simulink model "SIL_CessnaC172"  (R2021b)
settings: Solver=FixedStepAuto  StartTime=0  StopTime=T  FixedStep=0.01  RelTol=1e-3  EnableMultiTasking=on
model workspace (MAT data in the model file):
  SL_ROS_VariableLengthArrays_MaxSizes.CommonInfo.ArrayTruncateAction = 'EmitWarning'
  SL_ROS_VariableLengthArrays_MaxSizes.MsgTypeMap = containers.Map
  SL_ROS_VariableLengthArrays_MaxSizes.MsgTypeMap.serialization.keys = {'aircraft_communication/NetworkComm', 'aircraft_messages/Communication', 'aircraft_messages/NetworkComm', 'sensor_msgs/Image'}
  SL_ROS_VariableLengthArrays_MaxSizes.MsgTypeMap.serialization.values{1}.PropertyName = 'Comms'
  SL_ROS_VariableLengthArrays_MaxSizes.MsgTypeMap.serialization.values{1}.DataType = 'aircraft_communication/Communication'
  SL_ROS_VariableLengthArrays_MaxSizes.MsgTypeMap.serialization.values{1}.MaxLength = 4
  SL_ROS_VariableLengthArrays_MaxSizes.MsgTypeMap.serialization.values{2}.PropertyName = 'Ssid'
  SL_ROS_VariableLengthArrays_MaxSizes.MsgTypeMap.serialization.values{2}.DataType = 'uint8'
  SL_ROS_VariableLengthArrays_MaxSizes.MsgTypeMap.serialization.values{2}.MaxLength = 6
  SL_ROS_VariableLengthArrays_MaxSizes.MsgTypeMap.serialization.values{3}.PropertyName = 'Comms'
  SL_ROS_VariableLengthArrays_MaxSizes.MsgTypeMap.serialization.values{3}.DataType = 'aircraft_messages/Communication'
  SL_ROS_VariableLengthArrays_MaxSizes.MsgTypeMap.serialization.values{3}.MaxLength = 4
  SL_ROS_VariableLengthArrays_MaxSizes.MsgTypeMap.serialization.values{4}(1).PropertyName = 'Data'
  SL_ROS_VariableLengthArrays_MaxSizes.MsgTypeMap.serialization.values{4}(1).DataType = 'uint8'
  SL_ROS_VariableLengthArrays_MaxSizes.MsgTypeMap.serialization.values{4}(1).MaxLength = 259200
  SL_ROS_VariableLengthArrays_MaxSizes.MsgTypeMap.serialization.values{4}(2).PropertyName = 'Encoding'
  SL_ROS_VariableLengthArrays_MaxSizes.MsgTypeMap.serialization.values{4}(2).DataType = 'uint8'
  SL_ROS_VariableLengthArrays_MaxSizes.MsgTypeMap.serialization.values{4}(2).MaxLength = 259200
  SL_ROS_VariableLengthArrays_MaxSizes.MsgTypeMap.serialization.uniformity = 0
  SL_ROS_VariableLengthArrays_MaxSizes.MsgTypeMap.serialization.keyType = 'char'
  SL_ROS_VariableLengthArrays_MaxSizes.MsgTypeMap.serialization.valueType = 'any'
values from neighbouring files (symbols this model uses):
  airspeed_ref = 42    [start_Cessna172.m]
  altitude_ref = 300    [start_Cessna172.m]
  N_Waypoints = size(Waypoints,1)    [start_Cessna172.m]
  radius_waypoint = 200    [start_Cessna172.m]
  Waypoints = [1000 -1000 ... (first row only)    [start_Cessna172.m]
undefined symbols (not defined in the file or in its folder): Elevators, Propeller, RightAileron, RightFlap, Rudder
libraries: robotlib x7, slpidlib x3
settings Model: Creator=fcsou  LastModifiedBy=fabricio
settings SolverCC: AlgebraicLoopSolver=TrustRegion
settings OptimizationCC: EnhancedBackFolding=on  PassReuseOutputArgsThreshold=0  MaxStackSize=64  OptimizeBlockOrder=speed  DifferentSizesBufferReuse=on  OptimizationCustomize=off
settings DebuggingCC: ParameterTunabilityLossMsg=error  SFMachineParentedDataDiag=warning
settings HardwareCC: ProdBitPerPointer=32  ProdBitPerSizeT=32  ProdBitPerPtrDiffT=32  ProdLargestAtomicFloat=None  ProdIntDivRoundTo=Undefined  ProdEndianess=Unspecified  ProdWordSize=32  ProdHWDeviceType=Generic->Unspecified (assume 32-bit Generic)  UseEmbeddedCoderFeatures=off
settings SFSimCC: MATLABDynamicMemAlloc=off
settings RTWCC: Description=Embedded Coder  SystemTargetFile=ert.tlc  HardwareBoard=Robot Operating System (ROS)  TLCOptions="-aInlineSetEventsForThisBaseRateFcn=TLC_FALSE -aSuppressMultiTaskScheduler=TLC_FALSE  -aRateBasedStepFcn=0"  TemplateMakefile=ert_default_tmf  Toolchain=Catkin  TargetLang=C++
settings CodeAppCC: ForceParamTrailComments=on  OperatorAnnotations=on
settings ERTTargetCC: ERTCustomFileBanners=off  SupportContinuousTime=on  SupportNonInlinedSFcns=on  RemoveResetFunc=off  ModelStepFunctionPrototypeControlCompliant=off  ERTCustomFileTemplate=rostime_codertarget_file_process.tlc

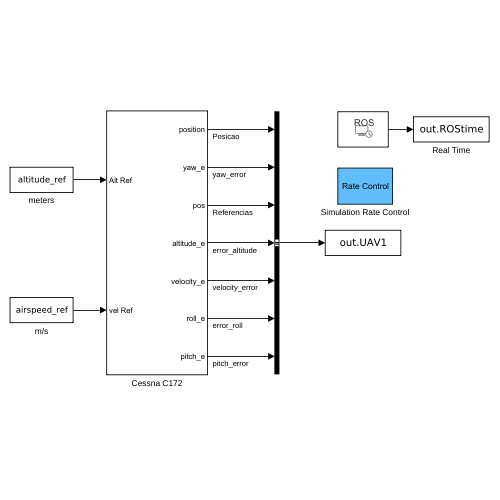
[thumbnail: Simulink's stored preview of the top-level diagram]
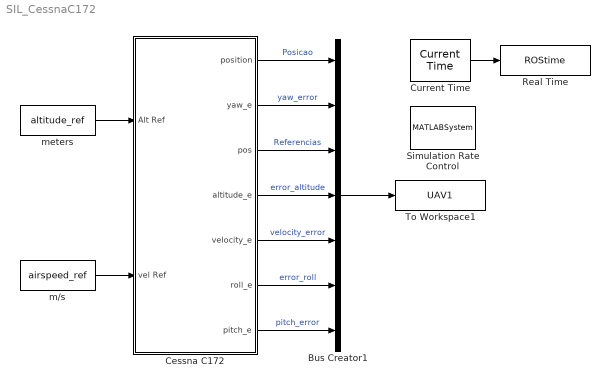
== system SIL_CessnaC172 ==
  Bus Creator1 : BusCreator  Inputs=7
  Cessna C172 : Subsystem
  Current Time : robotlib/Current Time  OutputFormat=double  SampleTime=-1  ModelName=SIL_CessnaC172
      settings: SourceProductBaseCode=RR
  Real Time : ToWorkspace  VariableName=ROStime  SaveFormat=Timeseries  SampleTime=-1
  Simulation Rate Control : MATLABSystem  System=ExampleHelperSimulationRateControl  SampleTime=0.01
      mask Type: ExampleHelperSimulationRateControl
      mask Display: disp('Rate Control');
  To Workspace1 : ToWorkspace  VariableName=UAV1  SaveFormat=Timeseries  SampleTime=-1
  m/s : Constant  Value=airspeed_ref
  meters : Constant  Value=altitude_ref
  wires:
  m/s/1 -> Cessna C172/2(vel Ref)
  meters/1 -> Cessna C172/1(Alt Ref)
  Bus Creator1/1 -> To Workspace1/1
  Current Time/1 -> Real Time/1
  Cessna C172/1(position) -> Bus Creator1/1  "Posicao"
  Cessna C172/2(yaw_e) -> Bus Creator1/2  "yaw_error"
  Cessna C172/3(pos) -> Bus Creator1/3  "Referencias"
  Cessna C172/4(altitude_e) -> Bus Creator1/4  "error_altitude"
  Cessna C172/5(velocity_e) -> Bus Creator1/5  "velocity_error"
  Cessna C172/6(roll_e) -> Bus Creator1/6  "error_roll"
  Cessna C172/7(pitch_e) -> Bus Creator1/7  "pitch_error"

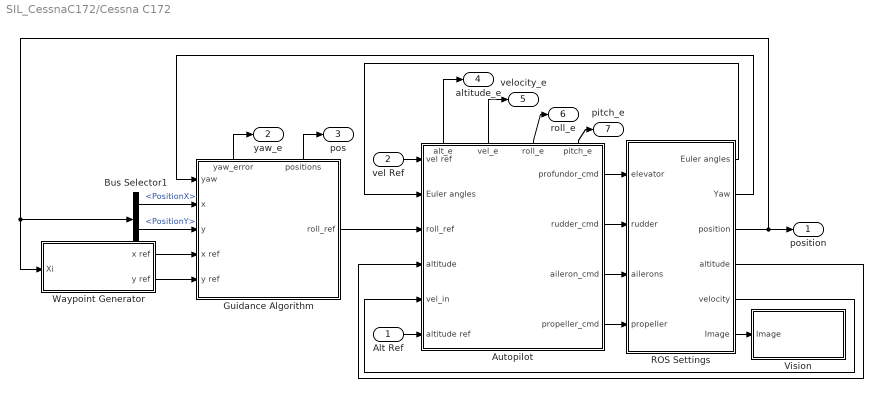
== system SIL_CessnaC172/Cessna C172 ==
  Alt Ref : Inport
  vel Ref : Inport  Port=2
  Autopilot : Subsystem
      settings: PortSchema="{\"entries\":[{\"content\":{\"sides\":[{\"content\":{\"connectorIds\":[\"In1\",\"In2\",\"In3\",\"In4\",\"In5\",\"In6\"]},\"type\":\"ConnectorPlacement.EquallySpacedRectSide\",\"uuid\":\"f5987fb5-26bd-460f-ada3-c62a2cc917d9\"},{\"content\":{\"connectorIds\":[\"Out1\",\"Out2\",\"Out3\",\"Out4\"],\"side\":\"RIGHT\"},\"type\":\"ConnectorPlacement.EquallySpacedRectSide\",\"uuid\":\"78b4fbb6-b2d6-45e8-a79e-ccfb1aa742fa\"},{\"content\":{\"connectorIds\":[\"Out5\",\"Out6\",\"Out7\",\"Out8\"],\"side\":\"TOP\"},\"type\":\"ConnectorPlacement.EquallySpacedRectSide\",\"uuid\":\"043ac8db-db42-42ba-ba46-d4f45f772f93\"},{\"content\":{\"connectorIds\":[],\"side\":\"HIDDEN\"},\"type\":\"ConnectorPlacement.EquallySpacedRectSide\",\"uuid\":\"557a5d68-6739-4613-818d-4b3751c4f08a\"}]},\"type\":\"ConnectorPlacement.EquallySpacedConnector\",\"uuid\":\"675ce67f-dd1b-4b16-8fb4-2c0be5e81414\"}],\"packageUris\":[\"http://schema.mathworks.com/mf0/Connector/R2020b\"],\"version\":\"1.0\"}"
  Bus Selector1 : BusSelector  OutputSignals=PositionX,PositionY
  Guidance Algorithm : Subsystem
      settings: PortSchema="{\"entries\":[{\"content\":{\"sides\":[{\"content\":{\"connectorIds\":[\"In1\",\"In2\",\"In3\",\"In4\",\"In5\"]},\"type\":\"ConnectorPlacement.EquallySpacedRectSide\",\"uuid\":\"b0b83658-dc10-4011-a234-ab17b261f867\"},{\"content\":{\"connectorIds\":[\"Out1\"],\"side\":\"RIGHT\"},\"type\":\"ConnectorPlacement.EquallySpacedRectSide\",\"uuid\":\"f99dae16-3a0a-4b7a-a248-8f98f89ef8fb\"},{\"content\":{\"connectorIds\":[\"Out2\",\"Out3\"],\"side\":\"TOP\"},\"type\":\"ConnectorPlacement.EquallySpacedRectSide\",\"uuid\":\"275bc05e-c915-4930-a6d1-ba5a3a506250\"},{\"content\":{\"connectorIds\":[],\"side\":\"HIDDEN\"},\"type\":\"ConnectorPlacement.EquallySpacedRectSide\",\"uuid\":\"a071ce22-c6e1-49a1-b318-d26a8e8cfe9f\"}]},\"type\":\"ConnectorPlacement.EquallySpacedConnector\",\"uuid\":\"e0998603-dd40-4b43-8488-1ee2e7350a27\"}],\"packageUris\":[\"http://schema.mathworks.com/mf0/Connector/R2020b\"],\"version\":\"1.0\"}"
  ROS Settings : Subsystem
  Vision : Subsystem
  Waypoint Generator : Subsystem
  position : Outport
  yaw_e : Outport  Port=2
  pos : Outport  Port=3
  altitude_e : Outport  Port=4
  velocity_e : Outport  Port=5
  roll_e : Outport  Port=6
  pitch_e : Outport  Port=7
  wires:
  Bus Selector1/2 -> Guidance Algorithm/3(y)  "<PositionY>"
  Bus Selector1/1 -> Guidance Algorithm/2(x)  "<PositionX>"
  Autopilot/3(aileron_cmd) -> ROS Settings/3(ailerons)
  ROS Settings/1(Euler angles) -> Autopilot/2(Euler angles)
  Guidance Algorithm/1(roll_ref) -> Autopilot/3(roll_ref)
  Autopilot/1(profundor_cmd) -> ROS Settings/1(elevator)
  ROS Settings/3(position) -> position/1, Waypoint Generator/1(Xi), Bus Selector1/1
  ROS Settings/4(altitude) -> Autopilot/4(altitude)
  ROS Settings/5(velocity) -> Autopilot/5(vel_in)
  Alt Ref/1 -> Autopilot/6(altitude ref)
  ROS Settings/2(Yaw) -> Guidance Algorithm/1(yaw)
  Guidance Algorithm/2(yaw_error) -> yaw_e/1
  Guidance Algorithm/3(positions) -> pos/1
  Autopilot/5(alt_e) -> altitude_e/1
  Autopilot/6(vel_e) -> velocity_e/1
  vel Ref/1 -> Autopilot/1(vel ref)
  Autopilot/7(roll_e) -> roll_e/1
  Autopilot/2(rudder_cmd) -> ROS Settings/2(rudder)
  Autopilot/4(propeller_cmd) -> ROS Settings/4(propeller)
  Waypoint Generator/1(x ref) -> Guidance Algorithm/4(x ref)
  Waypoint Generator/2(y ref) -> Guidance Algorithm/5(y ref)
  Autopilot/8(pitch_e) -> pitch_e/1
  ROS Settings/6(Image) -> Vision/1(Image)

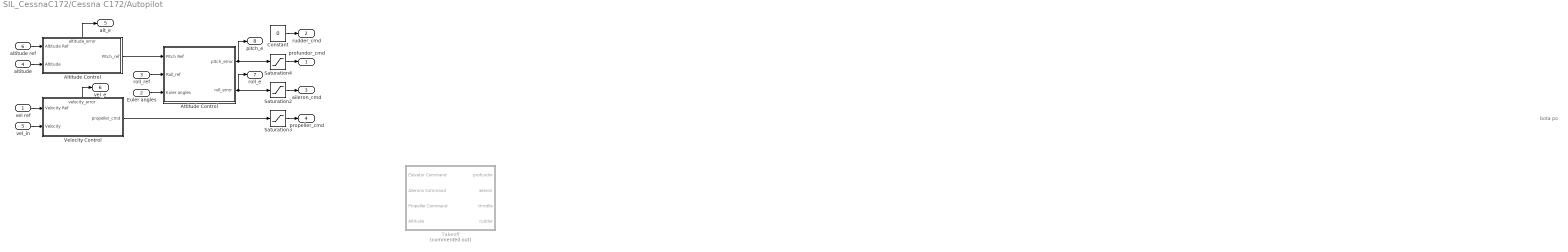
== system SIL_CessnaC172/Cessna C172/Autopilot ==
  note: bota po
  vel ref : Inport
  Euler angles : Inport  Port=2
  roll_ref : Inport  Port=3
  altitude : Inport  Port=4
  vel_in : Inport  Port=5
  altitude ref : Inport  Port=6
  Altitude Control : Subsystem
      settings: PortSchema="{\"entries\":[{\"content\":{\"sides\":[{\"content\":{\"connectorIds\":[\"In1\",\"In2\"]},\"type\":\"ConnectorPlacement.EquallySpacedRectSide\",\"uuid\":\"98c80c82-2588-492a-897d-d133440579b3\"},{\"content\":{\"connectorIds\":[\"Out1\"],\"side\":\"RIGHT\"},\"type\":\"ConnectorPlacement.EquallySpacedRectSide\",\"uuid\":\"157fcffb-564d-4941-a636-42e4165df758\"},{\"content\":{\"connectorIds\":[\"Out2\"],\"side\":\"TOP\"},\"type\":\"ConnectorPlacement.EquallySpacedRectSide\",\"uuid\":\"44b57248-226e-45fd-814c-d7eb072c2d1f\"},{\"content\":{\"connectorIds\":[],\"side\":\"HIDDEN\"},\"type\":\"ConnectorPlacement.EquallySpacedRectSide\",\"uuid\":\"dff6d6ab-ae11-4516-9107-00b7ae45fb5b\"}]},\"type\":\"ConnectorPlacement.EquallySpacedConnector\",\"uuid\":\"b6a62117-e3d4-4c2a-a3b5-b134a2ba950a\"}],\"packageUris\":[\"http://schema.mathworks.com/mf0/Connector/R2020b\"],\"version\":\"1.0\"}"
  Attitude Control : Subsystem
  Constant : Constant  Value=0
  Saturation2 : Saturate  UpperLimit=0.0523599  LowerLimit=-0.0523599
  Saturation3 : Saturate  UpperLimit=0.8  LowerLimit=0.6
  Saturation4 : Saturate  UpperLimit=0.0523599  LowerLimit=-0.0523599
  Takeoff : Subsystem  Commented=on
  Velocity Control : Subsystem
      settings: PortSchema="{\"entries\":[{\"content\":{\"sides\":[{\"content\":{\"connectorIds\":[\"In1\",\"In2\"]},\"type\":\"ConnectorPlacement.EquallySpacedRectSide\",\"uuid\":\"98c80c82-2588-492a-897d-d133440579b3\"},{\"content\":{\"connectorIds\":[\"Out1\"],\"side\":\"RIGHT\"},\"type\":\"ConnectorPlacement.EquallySpacedRectSide\",\"uuid\":\"157fcffb-564d-4941-a636-42e4165df758\"},{\"content\":{\"connectorIds\":[\"Out2\"],\"side\":\"TOP\"},\"type\":\"ConnectorPlacement.EquallySpacedRectSide\",\"uuid\":\"44b57248-226e-45fd-814c-d7eb072c2d1f\"},{\"content\":{\"connectorIds\":[],\"side\":\"HIDDEN\"},\"type\":\"ConnectorPlacement.EquallySpacedRectSide\",\"uuid\":\"dff6d6ab-ae11-4516-9107-00b7ae45fb5b\"}]},\"type\":\"ConnectorPlacement.EquallySpacedConnector\",\"uuid\":\"b6a62117-e3d4-4c2a-a3b5-b134a2ba950a\"}],\"packageUris\":[\"http://schema.mathworks.com/mf0/Connector/R2020b\"],\"version\":\"1.0\"}"
  profundor_cmd : Outport
  rudder_cmd : Outport  Port=2
  aileron_cmd : Outport  Port=3
  propeller_cmd : Outport  Port=4
  alt_e : Outport  Port=5
  vel_e : Outport  Port=6
  roll_e : Outport  Port=7
  pitch_e : Outport  Port=8
  wires:
  vel ref/1 -> Velocity Control/1(Velocity Ref)
  altitude ref/1 -> Altitude Control/1(Altitude Ref)
  vel_in/1 -> Velocity Control/2(Velocity)
  Altitude Control/2(altitude_error) -> alt_e/1
  Velocity Control/2(velocity_error) -> vel_e/1
  Altitude Control/1(Pitch_ref) -> Attitude Control/1(Pitch Ref)
  roll_ref/1 -> Attitude Control/2(Roll_ref)
  Euler angles/1 -> Attitude Control/3(Euler angles)
  Attitude Control/1(pitch_error) -> pitch_e/1, Saturation4/1
  Attitude Control/2(roll_error) -> Saturation2/1, roll_e/1
  Velocity Control/1(propeller_cmd) -> Saturation3/1
  Saturation3/1 -> propeller_cmd/1
  Saturation2/1 -> aileron_cmd/1
  Saturation4/1 -> profundor_cmd/1
  altitude/1 -> Altitude Control/2(Altitude)
  Constant/1 -> rudder_cmd/1

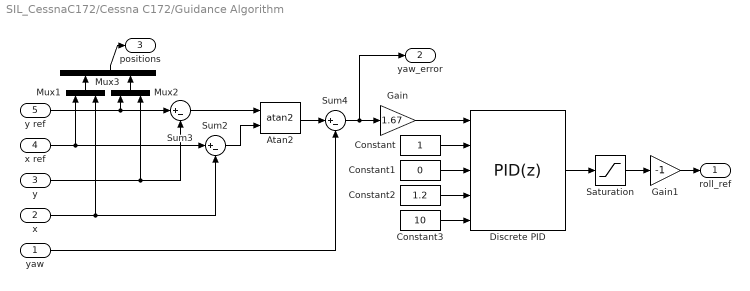
== system SIL_CessnaC172/Cessna C172/Guidance Algorithm ==
  yaw : Inport
  x : Inport  Port=2
  y : Inport  Port=3
  x ref : Inport  Port=4
  y ref : Inport  Port=5
  Atan2 : Trigonometry  Operator=atan2
  Constant : Constant
  Constant1 : Constant  Value=0
  Constant2 : Constant  Value=1.2
  Constant3 : Constant  Value=10
  Discrete PID : slpidlib/PID Controller  Controller=PID  Form=Parallel  TimeDomain=Discrete-time  UseExternalTs=off  SampleTime=-1  IntegratorMethod=Forward Euler  FilterMethod=Forward Euler  ControllerParametersSource=external  P=1  I=1  D=0  UseFilter=on  N=100  TunerSelectOption=Transfer Function Based (PID Tuner App)  InitialConditionSource=internal  InitialConditionForIntegrator=0  InitialConditionForFilter=0  DifferentiatorICPrevScaledInput=0  ExternalReset=none  TrackingMode=off  Kt=1  LimitOutput=off  SatLimitsSource=internal  UpperSaturationLimit=inf  LowerSaturationLimit=-inf  LinearizeAsGain=on  AntiWindupMode=none  Kb=1  POutMin=[]  POutMax=[]  IOutMin=[]  IOutMax=[]  DOutMin=[]  DOutMax=[]  NOutMin=[]  NOutMax=[]  SumOutMin=[]  SumOutMax=[]  SaturationOutMin=[]  SaturationOutMax=[]  PParamMin=[]  PParamMax=[]  IParamMin=[]  IParamMax=[]  DParamMin=[]  DParamMax=[]  NParamMin=[]  NParamMax=[]  KbParamMin=[]  KbParamMax=[]  KtParamMin=[]  KtParamMax=[]  KbOutMin=[]  KbOutMax=[]  KtOutMin=[]  KtOutMax=[]  IntegratorOutMin=[]  IntegratorOutMax=[]  FilterOutMin=[]  FilterOutMax=[]  SumI1OutMin=[]  SumI1OutMax=[]  SumI2OutMin=[]  SumI2OutMax=[]  SumI3OutMin=[]  SumI3OutMax=[]  SumI4OutMin=[]  SumI4OutMax=[]  SumDOutMin=[]  SumDOutMax=[]  DifferentiatorOutMin=[]  DifferentiatorOutMax=[]  FilterDiffOutCoefMin=[]  FilterDiffOutCoefMax=[]  ReciprocalOutMin=[]  ReciprocalOutMax=[]  SumDenOutMin=[]  SumDenOutMax=[]  SumNumOutMin=[]  SumNumOutMax=[]  DivideOutMin=[]  DivideOutMax=[]  UdiffTsProdOutMin=[]  UdiffTsProdOutMax=[]  NTsProdOutMin=[]  NTsProdOutMax=[]  UintegralTsProdOutMin=[]  UintegralTsProdOutMax=[]  UngainTsProdOutMin=[]  UngainTsProdOutMax=[]  IntegratorContinuousStateAttributes=''  IntegratorStateMustResolveToSignalObject=off  IntegratorRTWStateStorageClass=Auto  FilterContinuousStateAttributes=''  FilterStateMustResolveToSignalObject=off  FilterRTWStateStorageClass=Auto  ParallelPVariant=ExternalParameters  IdealPVariant=Disabled  IVariant=ExternalParameters  DVariant=ExternalParameters  IntegratorVariant=Discrete  SatVariant=Disabled  AWVariant=Passthrough  PCopyVariant=Disabled  TRVariant=Disabled  FdbkBlocksVariant=Forward  IdealPFdbkVariant=Disabled  SatFdbkVariant=Disabled  DerivativeFilterVariant=ForwardEulerFilter  NVariant=ExternalParameters  NCopyVariant=Disabled  FilterICVariant=InternalICsFilter  IntegratorICVariant=InternalICs  ExternalResetVariant=Disabled  TRSumVariant=Passthrough  SumFdbkVariant=Disabled  SumVariant=Sum_PID  TsampFilterVariant=InternalTs  TsampNgainVariant=Passthrough  TsampIntegralVariant=Passthrough  ExternalSaturationOutDataTypeStr=Inherit: Same as second input
  Gain : Gain  Gain=1.67
  Gain1 : Gain  Gain=-1
  Mux1 : Mux  Inputs=2
  Mux2 : Mux  Inputs=2
  Mux3 : Mux  Inputs=2
  Saturation : Saturate  UpperLimit=0.226893  LowerLimit=-0.226893
  Sum2 : Sum  Inputs=|+-
  Sum3 : Sum  Inputs=|+-
  Sum4 : Sum  Inputs=|+-
  roll_ref : Outport
  yaw_error : Outport  Port=2
  positions : Outport  Port=3
  wires:
  Mux1/1 -> Mux3/1
  Mux2/1 -> Mux3/2
  Saturation/1 -> Gain1/1
  Sum3/1 -> Atan2/1
  y/1 -> Sum3/2, Mux2/2
  y ref/1 -> Mux2/1, Sum3/1
  x ref/1 -> Mux1/1, Sum2/1
  x/1 -> Sum2/2, Mux1/2
  Sum2/1 -> Atan2/2
  Atan2/1 -> Sum4/1
  yaw/1 -> Sum4/2
  Mux3/1 -> positions/1
  Discrete PID/1 -> Saturation/1
  Sum4/1 -> Gain/1, yaw_error/1
  Gain1/1 -> roll_ref/1
  Constant/1 -> Discrete PID/2
  Constant1/1 -> Discrete PID/3
  Constant2/1 -> Discrete PID/4
  Constant3/1 -> Discrete PID/5
  Gain/1 -> Discrete PID/1

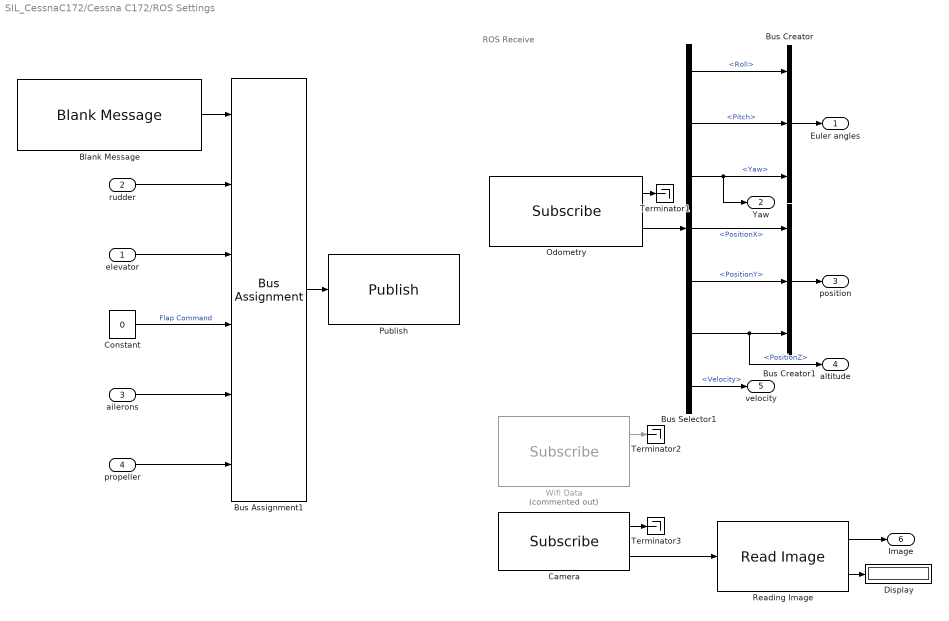
== system SIL_CessnaC172/Cessna C172/ROS Settings ==
  note: ROS Receive
  elevator : Inport
  rudder : Inport  Port=2
  ailerons : Inport  Port=3
  propeller : Inport  Port=4
  Blank Message : robotlib/Blank Message  messageClass=Message  entityType=cosmus_messages/Control_Surfaces  messageType=cosmus_messages/Control_Surfaces  SampleTime=-1  legacyBusStruct=off
  Bus Assignment1 : BusAssignment  AssignedSignals=Rudder,Elevators,RightFlap,RightAileron,Propeller
  Bus Creator : BusCreator  Inputs=3
  Bus Creator1 : BusCreator  Inputs=3
  Bus Selector1 : BusSelector  OutputSignals=Roll,Pitch,Yaw,PositionX,PositionY,PositionZ,Velocity
  Camera : robotlib/Subscribe  topicSource=Select from ROS network  topic=/uav1/camera/image_raw  messageType=sensor_msgs/Image  SampleTime=-1  legacyBusStruct=off  messageQueueLength=1
  Constant : Constant  Value=0
  Display : Display
  Odometry : robotlib/Subscribe  topicSource=Select from ROS network  topic=/uav1/ground_truth/Odometry  messageType=cosmus_communication/Odom  SampleTime=-1  legacyBusStruct=off  messageQueueLength=1
  Publish : robotlib/Publish  topicSource=Select from ROS network  topic=/uav1/command  messageType=cosmus_messages/Control_Surfaces  legacyBusStruct=off  messageQueueLength=1
  Reading Image : robotlib/Read Image  MaximumImageSize=[240, 360]  ImageEncoding=rgb8  ShowAlphaOutput=off  ShowErrorCodeOutput=on  VariableSizeOutputs=off
      settings: SourceProductBaseCode=RR
  Terminator1 : Terminator
  Terminator2 : Terminator
  Terminator3 : Terminator
  Wifi Data : robotlib/Subscribe  Commented=on  topicSource=Select from ROS network  topic=/uav1/wifi_receiver/data  messageType=cosmus_messages/NetworkComm  SampleTime=-1  legacyBusStruct=off  messageQueueLength=1
  Euler angles : Outport
  Yaw : Outport  Port=2
  position : Outport  Port=3
  altitude : Outport  Port=4
  velocity : Outport  Port=5
  Image : Outport  Port=6
  wires:
  Odometry/1 -> Terminator1/1
  Blank Message/1 -> Bus Assignment1/1
  Bus Selector1/3 -> Bus Creator/3, Yaw/1  "<Yaw>"
  Bus Creator/1 -> Euler angles/1
  Bus Selector1/1 -> Bus Creator/1  "<Roll>"
  Bus Selector1/2 -> Bus Creator/2  "<Pitch>"
  Constant/1 -> Bus Assignment1/4  "Flap Command"
  Bus Assignment1/1 -> Publish/1
  Odometry/2 -> Bus Selector1/1
  Bus Selector1/4 -> Bus Creator1/1  "<PositionX>"
  Bus Selector1/5 -> Bus Creator1/2  "<PositionY>"
  Bus Selector1/6 -> Bus Creator1/3, altitude/1  "<PositionZ>"
  propeller/1 -> Bus Assignment1/6
  ailerons/1 -> Bus Assignment1/5
  elevator/1 -> Bus Assignment1/3
  Bus Selector1/7 -> velocity/1  "<Velocity>"
  Bus Creator1/1 -> position/1
  rudder/1 -> Bus Assignment1/2
  Wifi Data/1 -> Terminator2/1
  Camera/2 -> Reading Image/1
  Reading Image/2 -> Display/1
  Reading Image/1 -> Image/1
  Camera/1 -> Terminator3/1

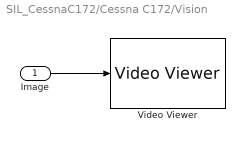
== system SIL_CessnaC172/Cessna C172/Vision ==
  Image : Inport
  Video Viewer : VideoViewer  FigPos=[1173 898 428 297]
  wires:
  Image/1 -> Video Viewer/1

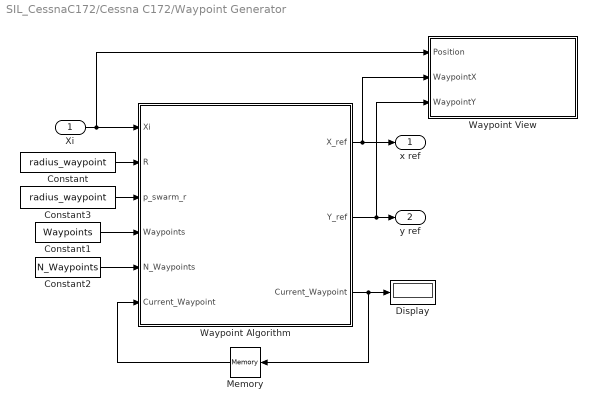
== system SIL_CessnaC172/Cessna C172/Waypoint Generator ==
  Xi : Inport
  Constant : Constant  Value=radius_waypoint
  Constant1 : Constant  Value=Waypoints
  Constant2 : Constant  Value=N_Waypoints
  Constant3 : Constant  Value=radius_waypoint
  Display : Display
  Memory : Memory
  Waypoint Algorithm : MATLAB Function  TreatAsAtomicUnit=on
  Waypoint View : MATLAB Function  TreatAsAtomicUnit=on
  x ref : Outport
  y ref : Outport  Port=2
  wires:
  Memory/1 -> Waypoint Algorithm/6("Current_Waypoint ")
  Constant1/1 -> Waypoint Algorithm/4(Waypoints)
  Xi/1 -> Waypoint View/1(Position), Waypoint Algorithm/1(Xi)
  Constant3/1 -> Waypoint Algorithm/3(p_swarm_r)
  Constant2/1 -> Waypoint Algorithm/5(N_Waypoints)
  Waypoint Algorithm/3(Current_Waypoint) -> Display/1, Memory/1
  Constant/1 -> Waypoint Algorithm/2(R)
  Waypoint Algorithm/1(X_ref) -> Waypoint View/2(WaypointX), x ref/1
  Waypoint Algorithm/2(Y_ref) -> Waypoint View/3(WaypointY), y ref/1

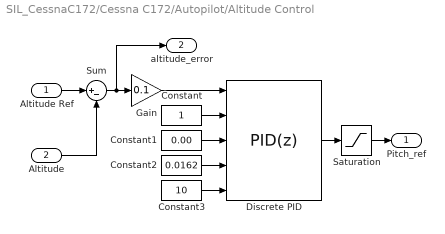
== system SIL_CessnaC172/Cessna C172/Autopilot/Altitude Control ==
  Altitude Ref : Inport
  Altitude : Inport  Port=2
  Constant : Constant
  Constant1 : Constant  Value=0.00
  Constant2 : Constant  Value=0.0162
  Constant3 : Constant  Value=10
  Discrete PID : slpidlib/PID Controller  Controller=PID  Form=Parallel  TimeDomain=Discrete-time  UseExternalTs=off  SampleTime=-1  IntegratorMethod=Forward Euler  FilterMethod=Forward Euler  ControllerParametersSource=external  P=1  I=1  D=0  UseFilter=on  N=100  TunerSelectOption=Transfer Function Based (PID Tuner App)  InitialConditionSource=internal  InitialConditionForIntegrator=0  InitialConditionForFilter=0  DifferentiatorICPrevScaledInput=0  ExternalReset=none  TrackingMode=off  Kt=1  LimitOutput=off  SatLimitsSource=internal  UpperSaturationLimit=inf  LowerSaturationLimit=-inf  LinearizeAsGain=on  AntiWindupMode=none  Kb=1  POutMin=[]  POutMax=[]  IOutMin=[]  IOutMax=[]  DOutMin=[]  DOutMax=[]  NOutMin=[]  NOutMax=[]  SumOutMin=[]  SumOutMax=[]  SaturationOutMin=[]  SaturationOutMax=[]  PParamMin=[]  PParamMax=[]  IParamMin=[]  IParamMax=[]  DParamMin=[]  DParamMax=[]  NParamMin=[]  NParamMax=[]  KbParamMin=[]  KbParamMax=[]  KtParamMin=[]  KtParamMax=[]  KbOutMin=[]  KbOutMax=[]  KtOutMin=[]  KtOutMax=[]  IntegratorOutMin=[]  IntegratorOutMax=[]  FilterOutMin=[]  FilterOutMax=[]  SumI1OutMin=[]  SumI1OutMax=[]  SumI2OutMin=[]  SumI2OutMax=[]  SumI3OutMin=[]  SumI3OutMax=[]  SumI4OutMin=[]  SumI4OutMax=[]  SumDOutMin=[]  SumDOutMax=[]  DifferentiatorOutMin=[]  DifferentiatorOutMax=[]  FilterDiffOutCoefMin=[]  FilterDiffOutCoefMax=[]  ReciprocalOutMin=[]  ReciprocalOutMax=[]  SumDenOutMin=[]  SumDenOutMax=[]  SumNumOutMin=[]  SumNumOutMax=[]  DivideOutMin=[]  DivideOutMax=[]  UdiffTsProdOutMin=[]  UdiffTsProdOutMax=[]  NTsProdOutMin=[]  NTsProdOutMax=[]  UintegralTsProdOutMin=[]  UintegralTsProdOutMax=[]  UngainTsProdOutMin=[]  UngainTsProdOutMax=[]  IntegratorContinuousStateAttributes=''  IntegratorStateMustResolveToSignalObject=off  IntegratorRTWStateStorageClass=Auto  FilterContinuousStateAttributes=''  FilterStateMustResolveToSignalObject=off  FilterRTWStateStorageClass=Auto  ParallelPVariant=ExternalParameters  IdealPVariant=Disabled  IVariant=ExternalParameters  DVariant=ExternalParameters  IntegratorVariant=Discrete  SatVariant=Disabled  AWVariant=Passthrough  PCopyVariant=Disabled  TRVariant=Disabled  FdbkBlocksVariant=Forward  IdealPFdbkVariant=Disabled  SatFdbkVariant=Disabled  DerivativeFilterVariant=ForwardEulerFilter  NVariant=ExternalParameters  NCopyVariant=Disabled  FilterICVariant=InternalICsFilter  IntegratorICVariant=InternalICs  ExternalResetVariant=Disabled  TRSumVariant=Passthrough  SumFdbkVariant=Disabled  SumVariant=Sum_PID  TsampFilterVariant=InternalTs  TsampNgainVariant=Passthrough  TsampIntegralVariant=Passthrough  ExternalSaturationOutDataTypeStr=Inherit: Same as second input
  Gain : Gain  Gain=0.1
  Saturation : Saturate  UpperLimit=0.78  LowerLimit=-0.78
  Sum : Sum  Inputs=|+-
  Pitch_ref : Outport
  altitude_error : Outport  Port=2
  wires:
  Saturation/1 -> Pitch_ref/1
  Altitude Ref/1 -> Sum/1
  Altitude/1 -> Sum/2
  Sum/1 -> altitude_error/1, Gain/1
  Constant/1 -> Discrete PID/2
  Constant1/1 -> Discrete PID/3
  Constant2/1 -> Discrete PID/4
  Constant3/1 -> Discrete PID/5
  Discrete PID/1 -> Saturation/1
  Gain/1 -> Discrete PID/1

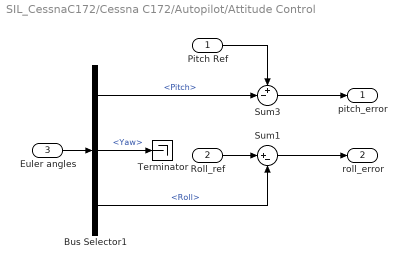
== system SIL_CessnaC172/Cessna C172/Autopilot/Attitude Control ==
  Pitch Ref : Inport
  Roll_ref : Inport  Port=2
  Euler angles : Inport  Port=3
  Bus Selector1 : BusSelector  OutputSignals=Pitch,Yaw,Roll
  Sum1 : Sum  Inputs=|+-
  Sum3 : Sum  Inputs=+-|
  Terminator : Terminator
  pitch_error : Outport
  roll_error : Outport  Port=2
  wires:
  Euler angles/1 -> Bus Selector1/1
  Sum1/1 -> roll_error/1
  Sum3/1 -> pitch_error/1
  Roll_ref/1 -> Sum1/1
  Bus Selector1/1 -> Sum3/2  "<Pitch>"
  Pitch Ref/1 -> Sum3/1
  Bus Selector1/3 -> Sum1/2  "<Roll>"
  Bus Selector1/2 -> Terminator/1  "<Yaw>"

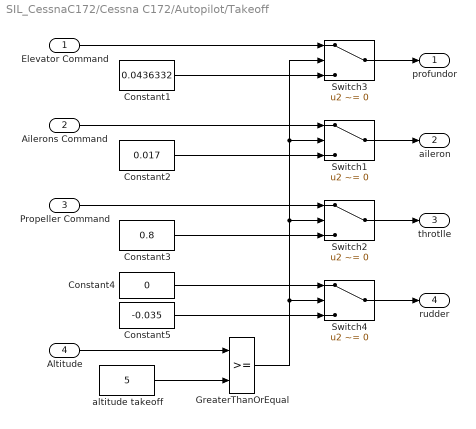
== system SIL_CessnaC172/Cessna C172/Autopilot/Takeoff ==
  Elevator Command : Inport
  Ailerons Command : Inport  Port=2
  Propeller Command : Inport  Port=3
  Altitude : Inport  Port=4
  Constant1 : Constant  Value=0.0436332
  Constant2 : Constant  Value=0.017
  Constant3 : Constant  Value=0.8
  Constant4 : Constant  Value=0
  Constant5 : Constant  Value=-0.035
  GreaterThanOrEqual : RelationalOperator  OutDataTypeStr=boolean  RndMeth=Simplest
  Switch{1..4} (4 alike) : Switch  Criteria=u2 ~= 0
  altitude takeoff : Constant  Value=5
  profundor : Outport
  aileron : Outport  Port=2
  throtlle : Outport  Port=3
  rudder : Outport  Port=4
  wires:
  Elevator Command/1 -> Switch3/1
  Switch3/1 -> profundor/1
  Ailerons Command/1 -> Switch1/1
  Switch1/1 -> aileron/1
  Switch2/1 -> throtlle/1
  Propeller Command/1 -> Switch2/1
  Constant1/1 -> Switch3/3
  Constant2/1 -> Switch1/3
  Constant3/1 -> Switch2/3
  altitude takeoff/1 -> GreaterThanOrEqual/2
  Altitude/1 -> GreaterThanOrEqual/1
  GreaterThanOrEqual/1 -> Switch4/2, Switch3/2, Switch1/2, Switch2/2
  Constant4/1 -> Switch4/1
  Constant5/1 -> Switch4/3
  Switch4/1 -> rudder/1

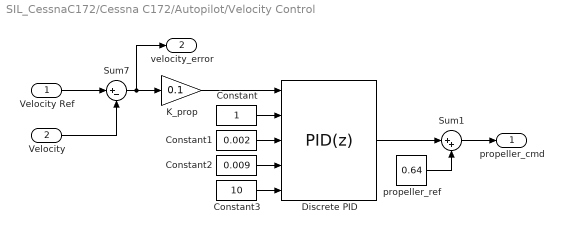
== system SIL_CessnaC172/Cessna C172/Autopilot/Velocity Control ==
  Velocity Ref : Inport
  Velocity : Inport  Port=2
  Constant : Constant
  Constant1 : Constant  Value=0.002
  Constant2 : Constant  Value=0.009
  Constant3 : Constant  Value=10
  Discrete PID : slpidlib/PID Controller  Controller=PID  Form=Parallel  TimeDomain=Discrete-time  UseExternalTs=off  SampleTime=-1  IntegratorMethod=Forward Euler  FilterMethod=Forward Euler  ControllerParametersSource=external  P=1  I=1  D=0  UseFilter=on  N=100  TunerSelectOption=Transfer Function Based (PID Tuner App)  InitialConditionSource=internal  InitialConditionForIntegrator=0  InitialConditionForFilter=0  DifferentiatorICPrevScaledInput=0  ExternalReset=none  TrackingMode=off  Kt=1  LimitOutput=off  SatLimitsSource=internal  UpperSaturationLimit=inf  LowerSaturationLimit=-inf  LinearizeAsGain=on  AntiWindupMode=none  Kb=1  POutMin=[]  POutMax=[]  IOutMin=[]  IOutMax=[]  DOutMin=[]  DOutMax=[]  NOutMin=[]  NOutMax=[]  SumOutMin=[]  SumOutMax=[]  SaturationOutMin=[]  SaturationOutMax=[]  PParamMin=[]  PParamMax=[]  IParamMin=[]  IParamMax=[]  DParamMin=[]  DParamMax=[]  NParamMin=[]  NParamMax=[]  KbParamMin=[]  KbParamMax=[]  KtParamMin=[]  KtParamMax=[]  KbOutMin=[]  KbOutMax=[]  KtOutMin=[]  KtOutMax=[]  IntegratorOutMin=[]  IntegratorOutMax=[]  FilterOutMin=[]  FilterOutMax=[]  SumI1OutMin=[]  SumI1OutMax=[]  SumI2OutMin=[]  SumI2OutMax=[]  SumI3OutMin=[]  SumI3OutMax=[]  SumI4OutMin=[]  SumI4OutMax=[]  SumDOutMin=[]  SumDOutMax=[]  DifferentiatorOutMin=[]  DifferentiatorOutMax=[]  FilterDiffOutCoefMin=[]  FilterDiffOutCoefMax=[]  ReciprocalOutMin=[]  ReciprocalOutMax=[]  SumDenOutMin=[]  SumDenOutMax=[]  SumNumOutMin=[]  SumNumOutMax=[]  DivideOutMin=[]  DivideOutMax=[]  UdiffTsProdOutMin=[]  UdiffTsProdOutMax=[]  NTsProdOutMin=[]  NTsProdOutMax=[]  UintegralTsProdOutMin=[]  UintegralTsProdOutMax=[]  UngainTsProdOutMin=[]  UngainTsProdOutMax=[]  IntegratorContinuousStateAttributes=''  IntegratorStateMustResolveToSignalObject=off  IntegratorRTWStateStorageClass=Auto  FilterContinuousStateAttributes=''  FilterStateMustResolveToSignalObject=off  FilterRTWStateStorageClass=Auto  ParallelPVariant=ExternalParameters  IdealPVariant=Disabled  IVariant=ExternalParameters  DVariant=ExternalParameters  IntegratorVariant=Discrete  SatVariant=Disabled  AWVariant=Passthrough  PCopyVariant=Disabled  TRVariant=Disabled  FdbkBlocksVariant=Forward  IdealPFdbkVariant=Disabled  SatFdbkVariant=Disabled  DerivativeFilterVariant=ForwardEulerFilter  NVariant=ExternalParameters  NCopyVariant=Disabled  FilterICVariant=InternalICsFilter  IntegratorICVariant=InternalICs  ExternalResetVariant=Disabled  TRSumVariant=Passthrough  SumFdbkVariant=Disabled  SumVariant=Sum_PID  TsampFilterVariant=InternalTs  TsampNgainVariant=Passthrough  TsampIntegralVariant=Passthrough  ExternalSaturationOutDataTypeStr=Inherit: Same as second input
  K_prop : Gain  Gain=0.1
  Sum1 : Sum  Inputs=|++
  Sum7 : Sum  Inputs=|+-
  propeller_ref : Constant  Value=0.64
  propeller_cmd : Outport
  velocity_error : Outport  Port=2
  wires:
  Velocity/1 -> Sum7/2
  Velocity Ref/1 -> Sum7/1
  Sum7/1 -> velocity_error/1, K_prop/1
  Sum1/1 -> propeller_cmd/1
  propeller_ref/1 -> Sum1/2
  Constant3/1 -> Discrete PID/5
  Constant/1 -> Discrete PID/2
  Discrete PID/1 -> Sum1/1
  Constant1/1 -> Discrete PID/3
  K_prop/1 -> Discrete PID/1
  Constant2/1 -> Discrete PID/4

== matlab function SIL_CessnaC172/Cessna C172/Waypoint Generator/Waypoint Algorithm ==
  data: Xi input; R input; p_swarm_r input; Waypoints input; N_Waypoints input; X_ref output; Y_ref output; Current_Waypoint output; Current_Waypoint input
function [X_ref, Y_ref, Current_Waypoint] = Next_Waypoint(Xi, R, p_swarm_r, Waypoints, N_Waypoints, Current_Waypoint)

    X_ref = Waypoints(Current_Waypoint + 1, 1);
    Y_ref = Waypoints(Current_Waypoint + 1, 2);

    if ( is_visited(Xi, R, p_swarm_r, X_ref, Y_ref)  )
        Current_Waypoint = mod(Current_Waypoint + 1, N_Waypoints);
    else
        Current_Waypoint = mod(Current_Waypoint, N_Waypoints);
    end

end

function visited = is_visited(Xi, R, p_swarm_r, wp1_X,wp1_Y)
    visited = 0;
    N = size(Xi,2);
    
    for i=1:N
        % if the aircraft inter the communication range and acces the
        % waypoitn area
        if( sqrt( (Xi(1, 1) - Xi(1, i) )^2 +(Xi(2, 1) - Xi(2, i))^2) < p_swarm_r && sqrt( (wp1_X - Xi(1, i) )^2 +(wp1_Y - Xi(2, i))^2) < R )
            visited = 1;
            return
        end
    end
    
end

== matlab function SIL_CessnaC172/Cessna C172/Waypoint Generator/Waypoint View ==
  data: Position input; WaypointX input; WaypointY input
function plotLaser(Position, WaypointX,WaypointY)
coder.extrinsic('plot');
persistent p;
persistent w;
if isempty(p)
    hold on
    p = plot(WaypointX, WaypointY, 'ro', 'MarkerSize',15);
    w = plot(Position(1), Position(2), 'b*');
    hold off
    set(gca,'XLim', [-3000 3000], 'YLim', [-3000 3000]);
end
if ishandle(p)
    set(p, 'XData', WaypointX);
    set(p, 'YData', WaypointY);
    set(w, 'XData', Position(1));
    set(w, 'YData', Position(2));
    drawnow limitrate;
end
